simulink subsystem "POWER"  (R2024b)
settings: Solver=VariableStepAuto  StartTime=0.0  StopTime=10.0  RelTol=1e-3
settings Model: Creator=JesseJabezArendse  LastModifiedBy=JesseJabezArendse

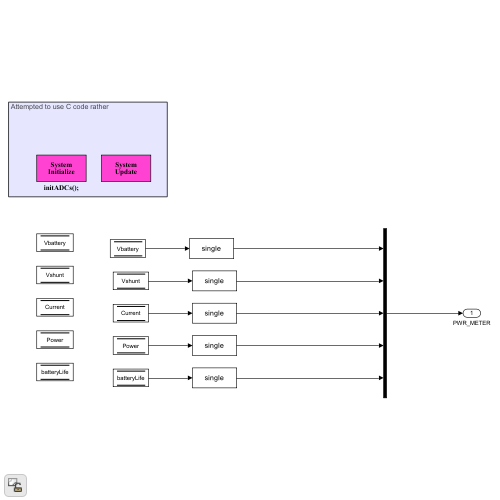
[thumbnail: Simulink's stored preview of the top-level diagram]
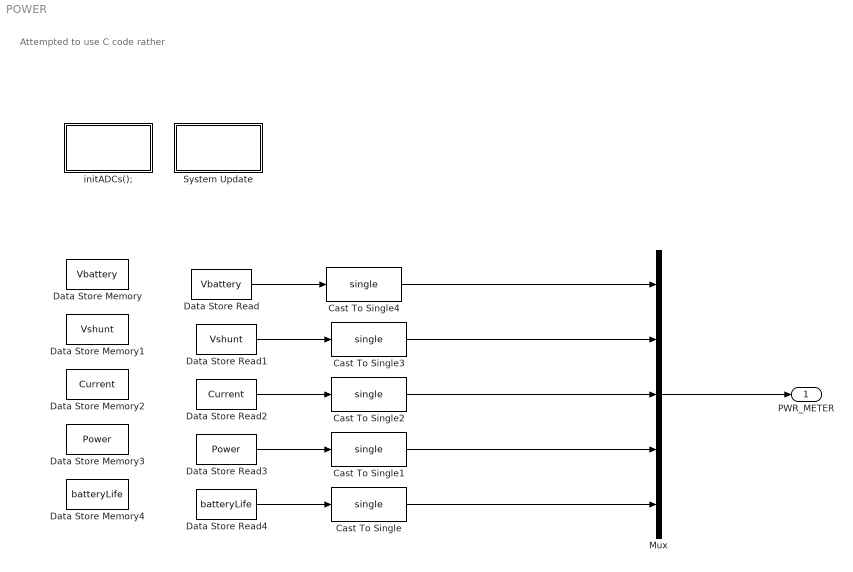
== system POWER ==
  note: Attempted to use C code rather
  Cast To Single{,1..4} (5 alike) : DataTypeConversion  OutDataTypeStr=single  SaturateOnIntegerOverflow=off  RndMeth=Floor
  Data Store Memory : DataStoreMemory  DataStoreName=Vbattery  WriteAfterWriteMsg=warning  ShowAdditionalParam=off  OutDataTypeStr=int16  Dimensions=1
  Data Store Memory1 : DataStoreMemory  DataStoreName=Vshunt  WriteAfterWriteMsg=warning  ShowAdditionalParam=off  OutDataTypeStr=int16  Dimensions=1
  Data Store Memory2 : DataStoreMemory  DataStoreName=Current  WriteAfterWriteMsg=warning  ShowAdditionalParam=off  OutDataTypeStr=int16  Dimensions=1
  Data Store Memory3 : DataStoreMemory  DataStoreName=Power  WriteAfterWriteMsg=warning  ShowAdditionalParam=off  OutDataTypeStr=int16  Dimensions=1
  Data Store Memory4 : DataStoreMemory  DataStoreName=batteryLife  WriteAfterWriteMsg=warning  ShowAdditionalParam=off  OutDataTypeStr=uint8  Dimensions=1
  Data Store Read : DataStoreRead  DataStoreName=Vbattery  IndexOptions=Index vector (dialog)  Indices=1  OutputSizes=1
  Data Store Read1 : DataStoreRead  DataStoreName=Vshunt  IndexOptions=Index vector (dialog)  Indices=1  OutputSizes=1
  Data Store Read2 : DataStoreRead  DataStoreName=Current  IndexOptions=Index vector (dialog)  Indices=1  OutputSizes=1
  Data Store Read3 : DataStoreRead  DataStoreName=Power  IndexOptions=Index vector (dialog)  Indices=1  OutputSizes=1
  Data Store Read4 : DataStoreRead  DataStoreName=batteryLife  IndexOptions=Index vector (dialog)  Indices=1  OutputSizes=1
  Mux : Mux  Inputs=5
  System Update : Subsystem  mask(System Update){ShowInLibBrowser=0}
      mask prompts: ShowInLibBrowser "Simulink:masks:CustCodeMaskParam1_MP"
      settings: CopyFcn=cccopyfcn(gcb)  OpenFcn=ccopenfcn('System Update Function')
      mask Help: eval('feval(''rtwprivate'',''rtwhelpview'',''rtw_sys_update_block'')');
      mask Display: disp('System\nUpdate');
  initADCs(); : Subsystem  mask(System Initialize){ShowInLibBrowser=0}
      mask prompts: ShowInLibBrowser "Simulink:masks:CustCodeMaskParam1_MP"
      settings: CopyFcn=cccopyfcn(gcb)  OpenFcn=ccopenfcn('System Initialize Function')
      mask Help: eval('feval(''rtwprivate'',''rtwhelpview'',''rtw_sys_initialize_block'')');
      mask Display: disp('System\nInitialize');
  PWR_METER : Outport
  wires:
  Data Store Read/1 -> Cast To Single4/1
  Data Store Read4/1 -> Cast To Single/1
  Data Store Read1/1 -> Cast To Single3/1
  Cast To Single2/1 -> Mux/3
  Cast To Single1/1 -> Mux/4
  Cast To Single3/1 -> Mux/2
  Cast To Single/1 -> Mux/5
  Cast To Single4/1 -> Mux/1
  Data Store Read2/1 -> Cast To Single2/1
  Data Store Read3/1 -> Cast To Single1/1
  Mux/1 -> PWR_METER/1

== system POWER/System Update ==

== system POWER/initADCs(); ==
